simulink subsystem "WiW2025DCSub"  (R2024b)
settings: Solver=VariableStepAuto  StartTime=0.0  StopTime=10.0  RelTol=1e-3
values from neighbouring files (symbols this model uses):
  parDC =     [parDC5MW.mat]
undefined symbols (not defined in the file or in its folder): DiscIntNeverNeededParam
settings Model: Creator=jb  LastModifiedBy=jb

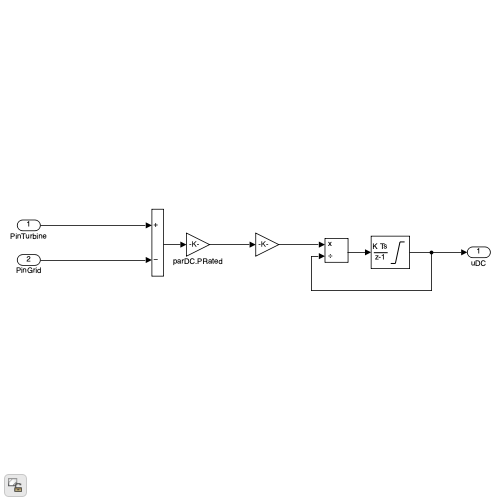
[thumbnail: Simulink's stored preview of the top-level diagram]
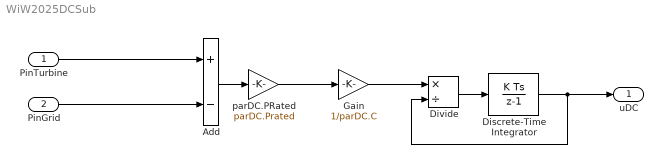
== system WiW2025DCSub ==
  PinTurbine : Inport
  PinGrid : Inport  Port=2
  Add : Sum  Inputs=+-
  Discrete-Time Integrator : DiscreteIntegrator  InitialCondition=parDC.uDC0  SampleTime=-1  LimitOutput=on  LowerSaturationLimit=100  ICPrevOutput=DiscIntNeverNeededParam  ICPrevScaledInput=DiscIntNeverNeededParam
  Divide : Product  Inputs=*/
  Gain : Gain  Gain=1/parDC.C
  parDC.PRated : Gain  Gain=parDC.Prated
  uDC : Outport
  wires:
  Add/1 -> parDC.PRated/1
  Divide/1 -> Discrete-Time Integrator/1
  PinTurbine/1 -> Add/1
  Gain/1 -> Divide/1
  PinGrid/1 -> Add/2
  parDC.PRated/1 -> Gain/1
  Discrete-Time Integrator/1 -> uDC/1, Divide/2
